simulink model "Fork_lift_traction_example_MMD"  (R2016a)
settings: Solver=ode45  StartTime=0.0  StopTime=100  RelTol=1e-3
libraries: simulink x1
settings Model: Creator=tammik2  LastModifiedBy=tammik2
settings DataIOCC: LimitDataPoints=on  SaveFormat=Array
settings HardwareCC: ProdBitPerPointer=32  ProdLargestAtomicFloat=None  ProdIntDivRoundTo=Undefined  ProdEndianess=Unspecified  ProdWordSize=32  ProdHWDeviceType=32-bit Generic
settings ModelReferenceCC: PropagateSignalLabelsOutOfModel=off
settings ConfigComp: CovModelRefEnable=Off

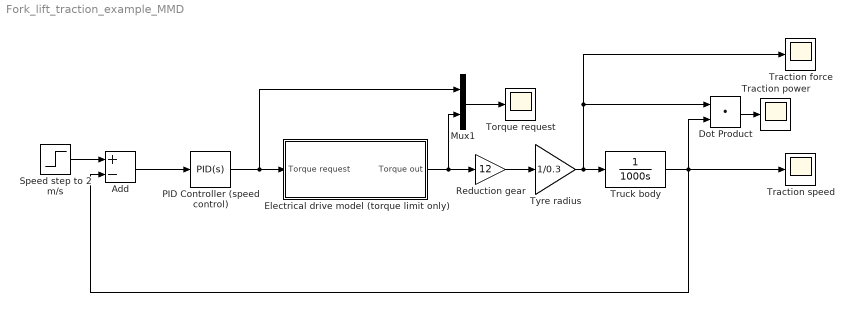
== system Fork_lift_traction_example_MMD ==
  Add : Sum  Inputs=+-
  Dot Product : DotProduct  InputSameDT=on  OutDataTypeStr=Inherit: Inherit via internal rule
  Electrical drive model (torque limit only) : Subsystem
  Mux1 : Mux  Inputs=2
  PID Controller (speed control) : simulink/Continuous/PID Controller  Controller=PID  TimeDomain=Continuous-time  SampleTime=-1  IntegratorMethod=Forward Euler  FilterMethod=Forward Euler  Form=Parallel  UseFilter=on  ControllerParametersSource=internal  P=25.690996042184  I=4.91423375667163  D=-5.4140291046049  N=1.72044274974478  InitialConditionSource=internal  InitialConditionForIntegrator=0  InitialConditionForFilter=0  ExternalReset=none  LimitOutput=off  UpperSaturationLimit=inf  LowerSaturationLimit=-inf  LinearizeAsGain=on  AntiWindupMode=none  Kb=1  TrackingMode=off  Kt=1  PParamMin=[]  PParamMax=[]  IParamMin=[]  IParamMax=[]  DParamMin=[]  DParamMax=[]  NParamMin=[]  NParamMax=[]  KbParamMin=[]  KbParamMax=[]  KtParamMin=[]  KtParamMax=[]  POutMin=[]  POutMax=[]  IOutMin=[]  IOutMax=[]  DOutMin=[]  DOutMax=[]  NOutMin=[]  NOutMax=[]  KbOutMin=[]  KbOutMax=[]  KtOutMin=[]  KtOutMax=[]  IntegratorOutMin=[]  IntegratorOutMax=[]  FilterOutMin=[]  FilterOutMax=[]  SumOutMin=[]  SumOutMax=[]  SumI1OutMin=[]  SumI1OutMax=[]  SumI2OutMin=[]  SumI2OutMax=[]  SumI3OutMin=[]  SumI3OutMax=[]  SumDOutMin=[]  SumDOutMax=[]  SaturationOutMin=[]  SaturationOutMax=[]  IntegratorContinuousStateAttributes=''  IntegratorStateMustResolveToSignalObject=off  IntegratorRTWStateStorageClass=Auto  FilterContinuousStateAttributes=''  FilterStateMustResolveToSignalObject=off  FilterRTWStateStorageClass=Auto  DifferentiatorICPrevScaledInput=0  DifferentiatorOutMin=[]  DifferentiatorOutMax=[]
  Reduction gear : Gain  Gain=12
  Speed step to 2 m/s : Step  After=2  SampleTime=0
  Torque request : Scope
  Traction force : Scope
  Traction power : Scope
  Traction speed : Scope
  Truck body : TransferFcn  Denominator="[1000  0]"
  Tyre radius : Gain  Gain=1/0.3
  wires:
  Speed step to 2 m/s/1 -> Add/1
  Reduction gear/1 -> Tyre radius/1
  Tyre radius/1 -> Traction force/1, Dot Product/1, Truck body/1
  Electrical drive model (torque limit only)/1(Torque out) -> Mux1/2, Reduction gear/1
  Dot Product/1 -> Traction power/1
  Truck body/1 -> Traction speed/1, Dot Product/2, Add/2
  Mux1/1 -> Torque request/1
  PID Controller (speed control)/1 -> Mux1/1, Electrical drive model (torque limit only)/1(Torque request)
  Add/1 -> PID Controller (speed control)/1

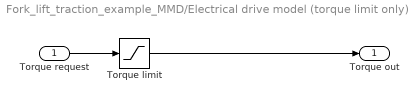
== system Fork_lift_traction_example_MMD/Electrical drive model (torque limit only) ==
  Torque request : Inport
  Torque limit : Saturate  UpperLimit=40  LowerLimit=-40
  Torque out : Outport
  wires:
  Torque request/1 -> Torque limit/1
  Torque limit/1 -> Torque out/1
